simulink model "if_else_action_subsystem"  (R2022a)
settings: Solver=VariableStepAuto  StartTime=0.0  StopTime=10.0  RelTol=1e-3
settings Model: Creator=Home computer  LastModifiedBy=Home computer

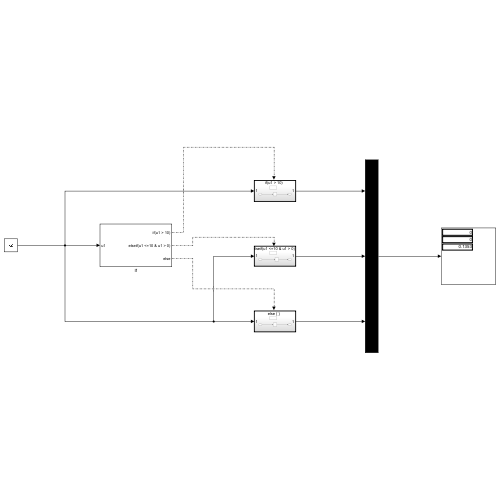
[thumbnail: Simulink's stored preview of the top-level diagram]
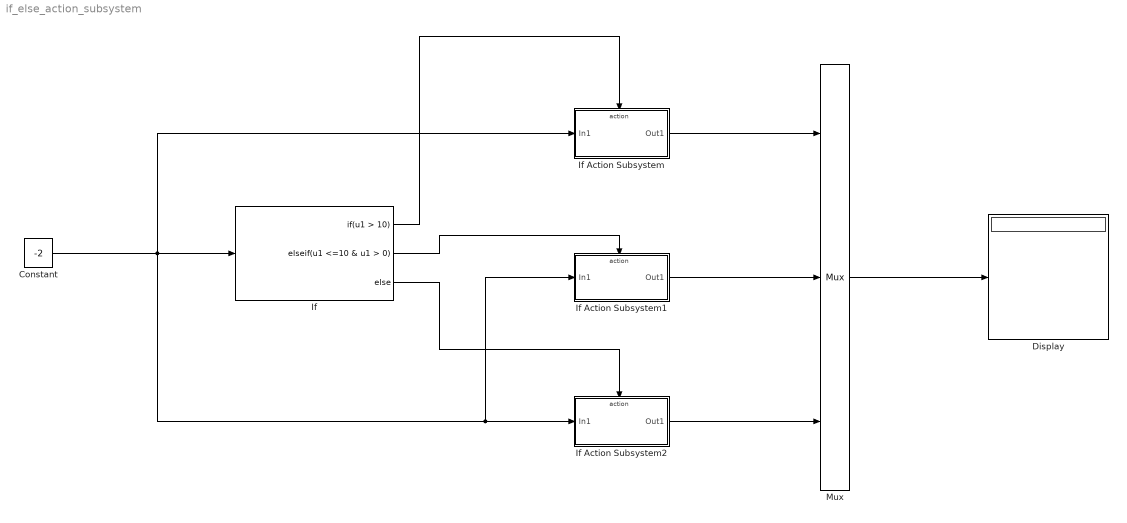
== system if_else_action_subsystem ==
  Constant : Constant  Value=-2
  Display : Display
  If : If  IfExpression=u1 > 10  ElseIfExpressions=u1 <=10 & u1 > 0
  If Action Subsystem : Subsystem  TreatAsAtomicUnit=on
  If Action Subsystem1 : Subsystem  TreatAsAtomicUnit=on
  If Action Subsystem2 : Subsystem  TreatAsAtomicUnit=on
  Mux : Mux  Inputs=3
  wires:
  If/1 -> If Action Subsystem/Action
  If/2 -> If Action Subsystem1/Action
  If/3 -> If Action Subsystem2/Action
  Constant/1 -> If Action Subsystem1/1(In1), If Action Subsystem2/1(In1), If/1, If Action Subsystem/1(In1)
  If Action Subsystem/1(Out1) -> Mux/1
  If Action Subsystem1/1(Out1) -> Mux/2
  If Action Subsystem2/1(Out1) -> Mux/3
  Mux/1 -> Display/1

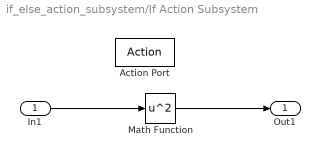
== system if_else_action_subsystem/If Action Subsystem ==
  In1 : Inport
  Action Port : ActionPort  ActionPortLabel=if(u1 > 10)
  Math Function : Math  Operator=square
  Out1 : Outport
  wires:
  In1/1 -> Math Function/1
  Math Function/1 -> Out1/1

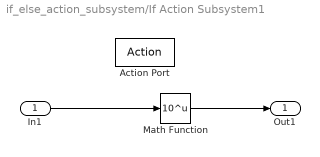
== system if_else_action_subsystem/If Action Subsystem1 ==
  In1 : Inport
  Action Port : ActionPort  ActionPortLabel=elseif(u1 <=10 & u1 > 0)
  Math Function : Math  Operator=10^u
  Out1 : Outport
  wires:
  In1/1 -> Math Function/1
  Math Function/1 -> Out1/1

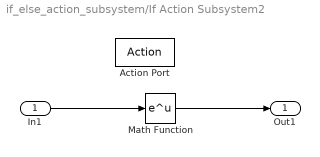
== system if_else_action_subsystem/If Action Subsystem2 ==
  In1 : Inport
  Action Port : ActionPort  ActionPortLabel=else
  Math Function : Math
  Out1 : Outport
  wires:
  In1/1 -> Math Function/1
  Math Function/1 -> Out1/1
